simulink model "CM010A_GmT1xxMcuCfg"  (R2013b)
settings: Solver=FixedStepDiscrete  SolverMode=SingleTasking  StartTime=0.0  StopTime=0.05  RelTol=1e-3
undefined symbols (not defined in the file): BATTVLTGSCAGFAC_ULS_F32, BATTVLTGSWD1SCAGFAC_ULS_F32, BATTVLTGSWD2SCAGFAC_ULS_F32, sigbuilder_block
libraries: CM010A_GmT1xxMcuCfg_ModelLibrary x68, simulink x31
(part 1 of 3)
settings Model: Creator=nz3zln  LastModifiedBy=wzvp6q
settings SolverCC: AutoInsertRateTranBlk=on
settings DataIOCC: SignalLoggingSaveFormat=ModelDataLogs
settings OptimizationCC: ExpressionDepthLimit=2147483647
settings DebuggingCC: FcnCallInpInsideContextMsg=UseLocalSettings  FrameProcessingCompatibilityMsg=error  StateNameClashWarn=warning
settings GRTTargetCC: CodeReplacementLibrary=C89/C90 (ANSI)  CombineOutputUpdateFcns=off  GRTInterface=on

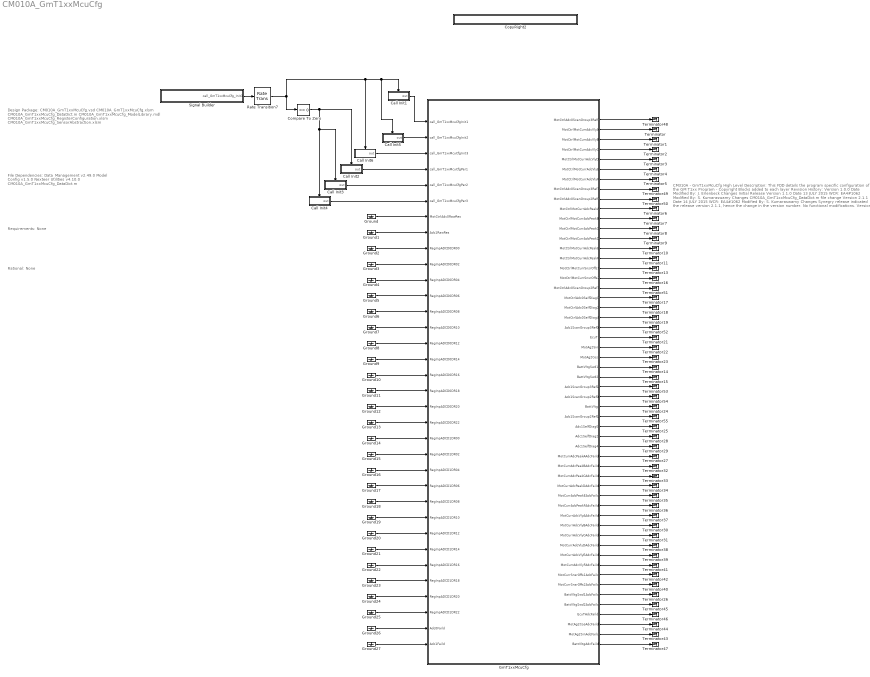
== system CM010A_GmT1xxMcuCfg ==
  note: File Dependencies:
      |
      | Data_Management v2.49.0
      | Model Config v1.5.0
      | Nexteer Utilities v4.10.0
      | CM010A_GmT1xxMcuCfg_DataDict.m
  note: CM310A - GmT1xxMcuCfg
      |
      | High Level Description:
      | This FDD details the program specific configuration of the GM T1xx Program
      |  - Copyright Blocks added to each layer
      |
      | Revision History:
      |
      | Version		1.0.0
      | Date
      | Modified By: 	J. Erlenbeck
      | Changes		Initial Release
      |
      | Version		1.1.0
      | Date 		13 JULY 2015
      | WCR:		EA4#1062
      | Modified By: 	S. Kumaraswamy
      | Changes		CM010A_GmT1xxMcuCfg_DataDict.m file change
      |
      | Version		2.1.1
      | Date 		14 JULY 2015
      | WCR:		EA4#1062
      | Modified By: 	S. Kumaraswamy
      | Changes		Synegry release indicated the release version 2.1.1, hence the
      | 			change in the version number. No functional modifications.
      |
      | Version		2.2.0
      | Date 		15 JULY 2015
      | WCR:		EA4#1109
      | Modified By: 	K. Patel
      | Changes		Motor Ag1 SPI DMA Trigger added to "CM010A_GmT1xxMcuCfg.xlsm"
      | Note: Timing vsd file need to be updated- current rev of FDD is not aligned with .vsd
      |
      |
      | Version		3.0.0
      | Date 		25JAN16
      | WCR:		EA4#3444
      | Modified By: 	Erlenbeck
      | Changes		Added GmT1xxMcuCfgPer3 to handle Adc failures
      |
      |
      | Version		3.3.0
      | Date 		07Jun16
      | WCR:		EA4#5916
      | Modified By: 	G. McCann
      | Changes		Add reference voltage read at start and end of Scan Groups 2 & 3
      |
      |
      | Version		3.4.0
      | Date 		13Sept16
      | WCR:		EA4#5916
      | Modified By: 	G. McCann
      | Changes		Removed MotCtrlAdc0DynRef and Adc1DynRef
      | 			Added NTCs in CM010A_GmT1xxMcuCfg.xlsm
      |
      |
      | Version		3.5.0
      | Date 		05Dec16
      | WCR:		EA4#8737
      | Modified By: 	G. McCann
      | Changes		No Model changes.
      | 			- Changed PwrTurnOffCtrl from PORT_PIN_LEVEL_HIGH to PORT_PIN_LEVEL_LOW
      | 			in CM010A_GmT1xxMcuCfg_PortConfig.xlsm
      | 			- Several changes to CM010A_GmT1xxMcuCfg_PortConfig.xlsm marked in red.
  note: Requirements:
      |
      | None
  note: Rational:
      |
      | None
  note: Design Package:
      |
      | CM010A_GmT1xxMcuCfg.vsd
      | CM010A_GmT1xxMcuCfg.xlsm
      | CM010A_GmT1xxMcuCfg_DataDict.m
      | CM010A_GmT1xxMcuCfg_ModelLibrary.mdl
      | CM010A_GmT1xxMcuCfg_RegisterConfiguration.xlsm
      | CM010A_GmT1xxMcuCfg_SensorAbstraction.xlsm
  Call Init1 : Subsystem  TreatAsAtomicUnit=on
  Call Init2 : Subsystem  TreatAsAtomicUnit=on
  Call Init3 : Subsystem  TreatAsAtomicUnit=on
  Call Init4 : Subsystem  TreatAsAtomicUnit=on
  Call Init5 : Subsystem  TreatAsAtomicUnit=on
  Call Init6 : Subsystem  TreatAsAtomicUnit=on
  Compare To Zero : simulink/Logic and Bit Operations/Compare To Zero  relop===  OutDataTypeStr=uint8
  CopyRight2 : Subsystem  Description=|  mask(Copyright Information){none=on}
      | Copyright info block.                                               
      |                                                                     
      | Place copyright information at the top of every subsystem in design.
      mask prompts: none "No parameters"
      mask help: Place copyright information at the top of every subsystem in design.
      mask Display:
      | NxtrConf = 'Nexteer Confidential';
      | 
      | sys = bdroot; %handle for the current model ("system")
      | first = get_param(sys,'Created');
      | first = first(end-3:end);  %year is last four digits
      | 
      | last = get_param(sys,'LastModifiedDate');
      | if isempty(last)
      |     last = datestr(now,'yyyy');
      | else
      |     last = last(end-3:end);
      | end
      | 
      | if strcmp(first,last)
      |     fprintf('%s -- Copyright %s Nexteer',NxtrConf,first)
      | else
      |     fprintf('%s -- %s%s- %s Nexteer',NxtrConf,char(169),first,last)
      | end
  GmT1xxMcuCfg : Subsystem
  Ground{,1..27} (28 alike) : Ground
  Rate Transition7 : RateTransition
  Signal Builder : Subsystem  Tag=STV Subsys  RequirementInfo={} %GIDa_2822100e_29fa_4197_9ccc_01864625f252  LoadFcn=sigbuilder_block('load');  StartFcn=sigbuilder_block('start');  StopFcn=sigbuilder_block('stop');  ClipboardFcn=sigbuilder_block('clipboard');  mask(Sigbuilder block){}
      mask help: Simulink:masks:SigbuilderBlock_MD
      mask init:
      | if ~strcmp(get_param(bdroot(gcbh),'SimulationStatus'),'stopped') tuvar = sigbuilder_block('maskInit'); end
      settings: CopyFcn=sigbuilder_block('copy');  DeleteFcn=sigbuilder_block('delete');  ModelCloseFcn=sigbuilder_block('modelClose');  PreSaveFcn=sigbuilder_block('preSave');  PauseFcn=sigbuilder_block('pause');  ContinueFcn=sigbuilder_block('continue');  NameChangeFcn=sigbuilder_block('namechange');  OpenFcn=sigbuilder_block('open',[61.5 32.25 865.5 462.75 ]);  CloseFcn=sigbuilder_block('close');
      mask Display: plot(0, 0, 100, 100,[2, 2, 32, 32, 2], [68, 8, 8, 68, 68],[32, 2], [38, 38], [32, 19, 2],[53, 60, 44], [32, 17, 17, 2],[16, 16, 31, 31]);txt = getActiveGroup(gcbh);text(2, 100, txt,'verticalAlignment', 'top');
  Terminator{,1..11,13..19,21..55} (54 alike) : Terminator
  wires:
  Signal Builder/1(call_GmT1xxMcuCfg_Init1) -> Rate Transition7/1
  Call Init1/1(out) -> GmT1xxMcuCfg/1(call_GmT1xxMcuCfgInit1)
  Rate Transition7/1 -> Compare To Zero/1, Call Init5/Enable, Call Init1/Enable, Call Init6/Enable
  Call Init2/1(out) -> GmT1xxMcuCfg/4(call_GmT1xxMcuCfgPer1)
  Call Init3/1(out) -> GmT1xxMcuCfg/5(call_GmT1xxMcuCfgPer2)
  Compare To Zero/1 -> Call Init4/Enable, Call Init3/Enable, Call Init2/Enable
  GmT1xxMcuCfg/2(MotCtrlMotCurrAdcVlyA) -> Terminator/1
  GmT1xxMcuCfg/3(MotCtrlMotCurrAdcVlyB) -> Terminator1/1
  GmT1xxMcuCfg/4(MotCtrlMotCurrAdcVlyC) -> Terminator2/1
  GmT1xxMcuCfg/5(MotCtrlMotCurrAdcVlyD) -> Terminator3/1
  GmT1xxMcuCfg/6(MotCtrlMotCurrAdcVlyE) -> Terminator4/1
  GmT1xxMcuCfg/7(MotCtrlMotCurrAdcVlyF) -> Terminator5/1
  GmT1xxMcuCfg/10(MotCtrlMotCurrAdcPeakA) -> Terminator6/1
  GmT1xxMcuCfg/11(MotCtrlMotCurrAdcPeakB) -> Terminator7/1
  GmT1xxMcuCfg/12(MotCtrlMotCurrAdcPeakC) -> Terminator8/1
  GmT1xxMcuCfg/13(MotCtrlMotCurrAdcPeakD) -> Terminator9/1
  GmT1xxMcuCfg/14(MotCtrlMotCurrAdcPeakE) -> Terminator10/1
  GmT1xxMcuCfg/15(MotCtrlMotCurrAdcPeakF) -> Terminator11/1
  GmT1xxMcuCfg/16(MotCtrlMotCurrSnsrOffs1) -> Terminator13/1
  GmT1xxMcuCfg/17(MotCtrlMotCurrSnsrOffs2) -> Terminator16/1
  GmT1xxMcuCfg/19(MotCtrlAdc0SelfDiag0) -> Terminator17/1
  GmT1xxMcuCfg/20(MotCtrlAdc0SelfDiag2) -> Terminator18/1
  GmT1xxMcuCfg/21(MotCtrlAdc0SelfDiag4) -> Terminator19/1
  GmT1xxMcuCfg/23(EcuT) -> Terminator21/1
  GmT1xxMcuCfg/24(MotAg2Sin) -> Terminator22/1
  GmT1xxMcuCfg/25(MotAg2Cos) -> Terminator23/1
  GmT1xxMcuCfg/26(BattVltgSwd1) -> Terminator14/1
  GmT1xxMcuCfg/27(BattVltgSwd2) -> Terminator15/1
  GmT1xxMcuCfg/30(BattVltg) -> Terminator24/1
  GmT1xxMcuCfg/32(Adc1SelfDiag0) -> Terminator25/1
  GmT1xxMcuCfg/33(Adc1SelfDiag2) -> Terminator28/1
  GmT1xxMcuCfg/34(Adc1SelfDiag4) -> Terminator29/1
  Ground23/1 -> GmT1xxMcuCfg/30(RegInpADCD1DR18)
  Ground20/1 -> GmT1xxMcuCfg/27(RegInpADCD1DR12)
  Ground21/1 -> GmT1xxMcuCfg/28(RegInpADCD1DR14)
  Ground16/1 -> GmT1xxMcuCfg/23(RegInpADCD1DR04)
  Ground22/1 -> GmT1xxMcuCfg/29(RegInpADCD1DR16)
  Ground19/1 -> GmT1xxMcuCfg/26(RegInpADCD1DR10)
  Ground17/1 -> GmT1xxMcuCfg/24(RegInpADCD1DR06)
  Ground18/1 -> GmT1xxMcuCfg/25(RegInpADCD1DR08)
  Ground6/1 -> GmT1xxMcuCfg/13(RegInpADCD0DR08)
  Ground1/1 -> GmT1xxMcuCfg/8(Adc1RawRes)
  Ground4/1 -> GmT1xxMcuCfg/11(RegInpADCD0DR04)
  Ground5/1 -> GmT1xxMcuCfg/12(RegInpADCD0DR06)
  Ground3/1 -> GmT1xxMcuCfg/10(RegInpADCD0DR02)
  Ground2/1 -> GmT1xxMcuCfg/9(RegInpADCD0DR00)
  Ground7/1 -> GmT1xxMcuCfg/14(RegInpADCD0DR10)
  Ground12/1 -> GmT1xxMcuCfg/19(RegInpADCD0DR20)
  Ground11/1 -> GmT1xxMcuCfg/18(RegInpADCD0DR18)
  Ground10/1 -> GmT1xxMcuCfg/17(RegInpADCD0DR16)
  Ground9/1 -> GmT1xxMcuCfg/16(RegInpADCD0DR14)
  Ground13/1 -> GmT1xxMcuCfg/20(RegInpADCD0DR22)
  Ground8/1 -> GmT1xxMcuCfg/15(RegInpADCD0DR12)
  Ground15/1 -> GmT1xxMcuCfg/22(RegInpADCD1DR02)
  Ground14/1 -> GmT1xxMcuCfg/21(RegInpADCD1DR00)
  Ground24/1 -> GmT1xxMcuCfg/31(RegInpADCD1DR20)
  Ground25/1 -> GmT1xxMcuCfg/32(RegInpADCD1DR22)
  Ground/1 -> GmT1xxMcuCfg/7(MotCtrlAdc0RawRes)
  GmT1xxMcuCfg/35(MotCurrAdcPeakAAdcFaild) -> Terminator27/1
  GmT1xxMcuCfg/36(MotCurrAdcPeakBAdcFaild) -> Terminator32/1
  GmT1xxMcuCfg/37(MotCurrAdcPeakCAdcFaild) -> Terminator33/1
  GmT1xxMcuCfg/38(MotCurrAdcPeakDAdcFaild) -> Terminator34/1
  GmT1xxMcuCfg/39(MotCurrAdcPeakEAdcFaild) -> Terminator35/1
  GmT1xxMcuCfg/40(MotCurrAdcPeakFAdcFaild) -> Terminator36/1
  GmT1xxMcuCfg/41(MotCurrAdcVlyAAdcFaild) -> Terminator37/1
  GmT1xxMcuCfg/42(MotCurrAdcVlyBAdcFaild) -> Terminator30/1
  GmT1xxMcuCfg/43(MotCurrAdcVlyCAdcFaild) -> Terminator31/1
  GmT1xxMcuCfg/44(MotCurrAdcVlyDAdcFaild) -> Terminator38/1
  GmT1xxMcuCfg/45(MotCurrAdcVlyEAdcFaild) -> Terminator39/1
  GmT1xxMcuCfg/46(MotCurrAdcVlyFAdcFaild) -> Terminator41/1
  GmT1xxMcuCfg/47(MotCurrSnsrOffs1AdcFaild) -> Terminator42/1
  GmT1xxMcuCfg/48(MotCurrSnsrOffs2AdcFaild) -> Terminator40/1
  GmT1xxMcuCfg/49(BattVltgSwd1AdcFaild) -> Terminator26/1
  GmT1xxMcuCfg/50(BattVltgSwd2AdcFaild) -> Terminator45/1
  GmT1xxMcuCfg/51(EcuTAdcFaild) -> Terminator46/1
  GmT1xxMcuCfg/52(MotAg2CosAdcFaild) -> Terminator44/1
  GmT1xxMcuCfg/53(MotAg2SinAdcFaild) -> Terminator43/1
  Ground26/1 -> GmT1xxMcuCfg/33(Adc0Faild)
  Ground27/1 -> GmT1xxMcuCfg/34(Adc1Faild)
  Call Init4/1(out) -> GmT1xxMcuCfg/6(call_GmT1xxMcuCfgPer3)
  Call Init5/1(out) -> GmT1xxMcuCfg/2(call_GmT1xxMcuCfgInit2)
  Call Init6/1(out) -> GmT1xxMcuCfg/3(call_GmT1xxMcuCfgInit3)
  GmT1xxMcuCfg/54(BattVltgAdcFaild) -> Terminator47/1
  GmT1xxMcuCfg/1(MotCtrlAdc0ScanGroup3Ref0) -> Terminator48/1
  GmT1xxMcuCfg/8(MotCtrlAdc0ScanGroup3Ref1) -> Terminator49/1
  GmT1xxMcuCfg/9(MotCtrlAdc0ScanGroup2Ref0) -> Terminator50/1
  GmT1xxMcuCfg/18(MotCtrlAdc0ScanGroup2Ref1) -> Terminator51/1
  GmT1xxMcuCfg/22(Adc1ScanGroup3Ref0) -> Terminator52/1
  GmT1xxMcuCfg/28(Adc1ScanGroup3Ref1) -> Terminator53/1
  GmT1xxMcuCfg/29(Adc1ScanGroup2Ref0) -> Terminator54/1
  GmT1xxMcuCfg/31(Adc1ScanGroup2Ref1) -> Terminator55/1

== system CM010A_GmT1xxMcuCfg/Call Init1 ==
  Enable : EnablePort
  Function Call Trigger : simulink/Ports & Subsystems/Function-Call Generator  RequirementInfo="{'linktype_rmi_doors' '000089e3 (/E-STEER_New/System Specification Documents/Core Specs/Subsystem Specs/System Functions FDD/SF-46  Gross Cross Check)' '#211' 'true' '3.1-1 The GCC function shall monitor every posted output motor comm' '' ; 'linktype_rmi_doors' '000089e3 (/E-STEER_New/System Specification Documents/Core Specs/Subsystem Specs/System Functions FDD/SF-46  Gross Cross Check)' '#182' 'true' '3.2.2-1 GCC shall be executed at a 0.002 second loop time.' '' } %GIDa_ff755a2e_49d1_45f7_8591_3ce0ef475338"  sample_time=0.0005  numberOfIterations=1
  out : Outport
  wires:
  Function Call Trigger/1 -> out/1

== system CM010A_GmT1xxMcuCfg/Call Init2 ==
  Enable : EnablePort
  Function Call Trigger : simulink/Ports & Subsystems/Function-Call Generator  RequirementInfo="{'linktype_rmi_doors' '000089e3 (/E-STEER_New/System Specification Documents/Core Specs/Subsystem Specs/System Functions FDD/SF-46  Gross Cross Check)' '#211' 'true' '3.1-1 The GCC function shall monitor every posted output motor comm' '' ; 'linktype_rmi_doors' '000089e3 (/E-STEER_New/System Specification Documents/Core Specs/Subsystem Specs/System Functions FDD/SF-46  Gross Cross Check)' '#182' 'true' '3.2.2-1 GCC shall be executed at a 0.002 second loop time.' '' } %GIDa_ba5be832_aeac_40ae_ae53_3fd25198366e"  sample_time=0.0005  numberOfIterations=1
  out : Outport
  wires:
  Function Call Trigger/1 -> out/1

== system CM010A_GmT1xxMcuCfg/Call Init3 ==
  Enable : EnablePort
  Function Call Trigger : simulink/Ports & Subsystems/Function-Call Generator  RequirementInfo="{'linktype_rmi_doors' '000089e3 (/E-STEER_New/System Specification Documents/Core Specs/Subsystem Specs/System Functions FDD/SF-46  Gross Cross Check)' '#211' 'true' '3.1-1 The GCC function shall monitor every posted output motor comm' '' ; 'linktype_rmi_doors' '000089e3 (/E-STEER_New/System Specification Documents/Core Specs/Subsystem Specs/System Functions FDD/SF-46  Gross Cross Check)' '#182' 'true' '3.2.2-1 GCC shall be executed at a 0.002 second loop time.' '' } %GIDa_bf682727_f4b1_4f52_ae72_c6f6d8d412d7"  sample_time=0.002  numberOfIterations=1
  out : Outport
  wires:
  Function Call Trigger/1 -> out/1

== system CM010A_GmT1xxMcuCfg/Call Init4 ==
  Enable : EnablePort
  Function Call Trigger : simulink/Ports & Subsystems/Function-Call Generator  RequirementInfo="{'linktype_rmi_doors' '000089e3 (/E-STEER_New/System Specification Documents/Core Specs/Subsystem Specs/System Functions FDD/SF-46  Gross Cross Check)' '#211' 'true' '3.1-1 The GCC function shall monitor every posted output motor comm' '' ; 'linktype_rmi_doors' '000089e3 (/E-STEER_New/System Specification Documents/Core Specs/Subsystem Specs/System Functions FDD/SF-46  Gross Cross Check)' '#182' 'true' '3.2.2-1 GCC shall be executed at a 0.002 second loop time.' '' } %GIDa_39162fcb_260a_4191_9640_bf2fa4fe87e2"  sample_time=0.002  numberOfIterations=1
  out : Outport
  wires:
  Function Call Trigger/1 -> out/1

== system CM010A_GmT1xxMcuCfg/Call Init5 ==
  Enable : EnablePort
  Function Call Trigger : simulink/Ports & Subsystems/Function-Call Generator  RequirementInfo="{'linktype_rmi_doors' '000089e3 (/E-STEER_New/System Specification Documents/Core Specs/Subsystem Specs/System Functions FDD/SF-46  Gross Cross Check)' '#211' 'true' '3.1-1 The GCC function shall monitor every posted output motor comm' '' ; 'linktype_rmi_doors' '000089e3 (/E-STEER_New/System Specification Documents/Core Specs/Subsystem Specs/System Functions FDD/SF-46  Gross Cross Check)' '#182' 'true' '3.2.2-1 GCC shall be executed at a 0.002 second loop time.' '' } %GIDa_52b82f2d_d21e_4ccf_9b87_2b660c433421"  sample_time=0.0005  numberOfIterations=1
  out : Outport
  wires:
  Function Call Trigger/1 -> out/1

== system CM010A_GmT1xxMcuCfg/Call Init6 ==
  Enable : EnablePort
  Function Call Trigger : simulink/Ports & Subsystems/Function-Call Generator  RequirementInfo="{'linktype_rmi_doors' '000089e3 (/E-STEER_New/System Specification Documents/Core Specs/Subsystem Specs/System Functions FDD/SF-46  Gross Cross Check)' '#211' 'true' '3.1-1 The GCC function shall monitor every posted output motor comm' '' ; 'linktype_rmi_doors' '000089e3 (/E-STEER_New/System Specification Documents/Core Specs/Subsystem Specs/System Functions FDD/SF-46  Gross Cross Check)' '#182' 'true' '3.2.2-1 GCC shall be executed at a 0.002 second loop time.' '' } %GIDa_40b20fc1_ef82_4ce8_9bb2_77ecb7477d85"  sample_time=0.0005  numberOfIterations=1
  out : Outport
  wires:
  Function Call Trigger/1 -> out/1

== system CM010A_GmT1xxMcuCfg/CopyRight2 ==

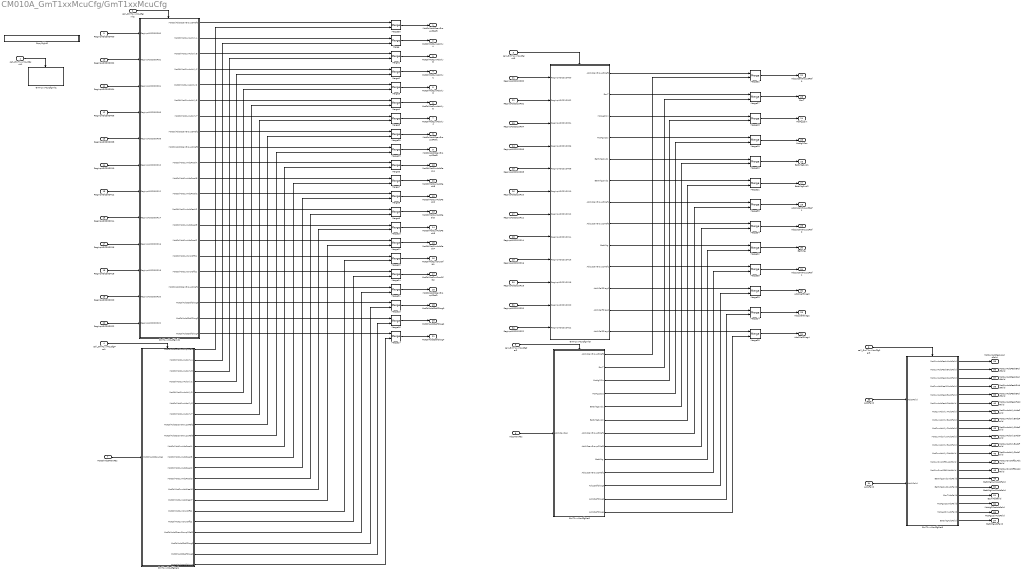
== system CM010A_GmT1xxMcuCfg/GmT1xxMcuCfg ==
  call_GmT1xxMcuCfgInit1 : Inport
  call_GmT1xxMcuCfgInit2 : Inport  Port=2
  call_GmT1xxMcuCfgInit3 : Inport  Port=3
  call_GmT1xxMcuCfgPer1 : Inport  Port=4
  call_GmT1xxMcuCfgPer2 : Inport  Port=5
  call_GmT1xxMcuCfgPer3 : Inport  Port=6
  MotCtrlAdc0RawRes : Inport  Port=7
  Adc1RawRes : Inport  Port=8
  RegInpADCD0DR00 : Inport  Port=9  OutDataTypeStr=uint32
  RegInpADCD0DR02 : Inport  Port=10  OutDataTypeStr=uint32
  RegInpADCD0DR04 : Inport  Port=11  OutDataTypeStr=uint32
  RegInpADCD0DR06 : Inport  Port=12  OutDataTypeStr=uint32
  RegInpADCD0DR08 : Inport  Port=13  OutDataTypeStr=uint32
  RegInpADCD0DR10 : Inport  Port=14  OutDataTypeStr=uint32
  RegInpADCD0DR12 : Inport  Port=15  OutDataTypeStr=uint32
  RegInpADCD0DR14 : Inport  Port=16  OutDataTypeStr=uint32
  RegInpADCD0DR16 : Inport  Port=17  OutDataTypeStr=uint32
  RegInpADCD0DR18 : Inport  Port=18  OutDataTypeStr=uint32
  RegInpADCD0DR20 : Inport  Port=19  OutDataTypeStr=uint32
  RegInpADCD0DR22 : Inport  Port=20  OutDataTypeStr=uint32
  RegInpADCD1DR00 : Inport  Port=21  OutDataTypeStr=uint32
  RegInpADCD1DR02 : Inport  Port=22  OutDataTypeStr=uint32
  RegInpADCD1DR04 : Inport  Port=23  OutDataTypeStr=uint32
  RegInpADCD1DR06 : Inport  Port=24  OutDataTypeStr=uint32
  RegInpADCD1DR08 : Inport  Port=25  OutDataTypeStr=uint32
  RegInpADCD1DR10 : Inport  Port=26  OutDataTypeStr=uint32
  RegInpADCD1DR12 : Inport  Port=27  OutDataTypeStr=uint32
  RegInpADCD1DR14 : Inport  Port=28  OutDataTypeStr=uint32
  RegInpADCD1DR16 : Inport  Port=29  OutDataTypeStr=uint32
  RegInpADCD1DR18 : Inport  Port=30  OutDataTypeStr=uint32
  RegInpADCD1DR20 : Inport  Port=31  OutDataTypeStr=uint32
  RegInpADCD1DR22 : Inport  Port=32  OutDataTypeStr=uint32
  Adc0Faild : Inport  Port=33
  Adc1Faild : Inport  Port=34
  CopyRight2 : Subsystem  Description=|  mask(Copyright Information){none=on}
      | Copyright info block.                                               
      |                                                                     
      | Place copyright information at the top of every subsystem in design.
      mask prompts: none "No parameters"
      mask help: Place copyright information at the top of every subsystem in design.
      mask Display:
      | NxtrConf = 'Nexteer Confidential';
      | 
      | sys = bdroot; %handle for the current model ("system")
      | first = get_param(sys,'Created');
      | first = first(end-3:end);  %year is last four digits
      | 
      | last = get_param(sys,'LastModifiedDate');
      | if isempty(last)
      |     last = datestr(now,'yyyy');
      | else
      |     last = last(end-3:end);
      | end
      | 
      | if strcmp(first,last)
      |     fprintf('%s -- Copyright %s Nexteer',NxtrConf,first)
      | else
      |     fprintf('%s -- %s%s- %s Nexteer',NxtrConf,char(169),first,last)
      | end
  GmT1xxMcuCfgInit1 : Subsystem
  GmT1xxMcuCfgInit2 : Subsystem
  GmT1xxMcuCfgInit3 : Subsystem
  GmT1xxMcuCfgPer1 : Subsystem  RequirementInfo={'linktype_rmi_doors' '0000c472 (/ESG Group/FDD Module Requirements/EA4 Specific/CM300A_Adc0CfgAndUse)' '#CM300A_76' 'true' 'REQ: CM300A_76' '' ; 'linktype_rmi_doors' '0000c472 (/ESG Group/FDD Module Requirements/EA4 Specific/CM300A_Adc0CfgAndUse)' '#CM300A_81' 'true' 'REQ: CM300A_81' '' ; 'linktype_rmi_doors' '0000c472 (/ESG Group/FDD Module Requirements/EA4 Specific/CM300A_Adc0CfgAndUse)' '#CM300A_82' 'true' 'REQ: CM300A_82' '' } %GIDa_873a1ca9_93ed_4591_b882_6d7fd3820ab2
      settings: AttributesFormatString=Priority: %<Priority>
  GmT1xxMcuCfgPer2 : Subsystem  RequirementInfo={'linktype_rmi_doors' '0000c472 (/ESG Group/FDD Module Requirements/EA4 Specific/CM300A_Adc0CfgAndUse)' '#CM300A_76' 'true' 'REQ: CM300A_76' '' ; 'linktype_rmi_doors' '0000c472 (/ESG Group/FDD Module Requirements/EA4 Specific/CM300A_Adc0CfgAndUse)' '#CM300A_81' 'true' 'REQ: CM300A_81' '' ; 'linktype_rmi_doors' '0000c472 (/ESG Group/FDD Module Requirements/EA4 Specific/CM300A_Adc0CfgAndUse)' '#CM300A_82' 'true' 'REQ: CM300A_82' '' } %GIDa_f8eec309_27b4_4df0_b18c_c2951f94362c
      settings: AttributesFormatString=Priority: %<Priority>
  GmT1xxMcuCfgPer3 : Subsystem  RequirementInfo={'linktype_rmi_doors' '0000c472 (/ESG Group/FDD Module Requirements/EA4 Specific/CM300A_Adc0CfgAndUse)' '#CM300A_76' 'true' 'REQ: CM300A_76' '' ; 'linktype_rmi_doors' '0000c472 (/ESG Group/FDD Module Requirements/EA4 Specific/CM300A_Adc0CfgAndUse)' '#CM300A_81' 'true' 'REQ: CM300A_81' '' ; 'linktype_rmi_doors' '0000c472 (/ESG Group/FDD Module Requirements/EA4 Specific/CM300A_Adc0CfgAndUse)' '#CM300A_82' 'true' 'REQ: CM300A_82' '' } %GIDa_f61b09d0_e9f4_4379_bee3_c878705b543d
      settings: AttributesFormatString=Priority: %<Priority>
  Merge{,1..11,13..25,27..35} (34 alike) : Merge
  MotCtrlAdc0ScanGroup3Ref0 : Outport
  MotCtrlMotCurrAdcVlyA : Outport  Port=2
  MotCtrlMotCurrAdcVlyB : Outport  Port=3
  MotCtrlMotCurrAdcVlyC : Outport  Port=4
  MotCtrlMotCurrAdcVlyD : Outport  Port=5
  MotCtrlMotCurrAdcVlyE : Outport  Port=6
  MotCtrlMotCurrAdcVlyF : Outport  Port=7
  MotCtrlAdc0ScanGroup3Ref1 : Outport  Port=8
  MotCtrlAdc0ScanGroup2Ref0 : Outport  Port=9
  MotCtrlMotCurrAdcPeakA : Outport  Port=10
  MotCtrlMotCurrAdcPeakB : Outport  Port=11
  MotCtrlMotCurrAdcPeakC : Outport  Port=12
  MotCtrlMotCurrAdcPeakD : Outport  Port=13
  MotCtrlMotCurrAdcPeakE : Outport  Port=14
  MotCtrlMotCurrAdcPeakF : Outport  Port=15
  MotCtrlMotCurrSnsrOffs1 : Outport  Port=16
  MotCtrlMotCurrSnsrOffs2 : Outport  Port=17
  MotCtrlAdc0ScanGroup2Ref1 : Outport  Port=18
  MotCtrlAdc0SelfDiag0 : Outport  Port=19
  MotCtrlAdc0SelfDiag2 : Outport  Port=20
  MotCtrlAdc0SelfDiag4 : Outport  Port=21
  Adc1ScanGroup3Ref0 : Outport  Port=22
  EcuT : Outport  Port=23
  MotAg2Sin : Outport  Port=24
  MotAg2Cos : Outport  Port=25
  BattVltgSwd1 : Outport  Port=26
  BattVltgSwd2 : Outport  Port=27
  Adc1ScanGroup3Ref1 : Outport  Port=28
  Adc1ScanGroup2Ref0 : Outport  Port=29
  BattVltg : Outport  Port=30
  Adc1ScanGroup2Ref1 : Outport  Port=31
  Adc1SelfDiag0 : Outport  Port=32
  Adc1SelfDiag2 : Outport  Port=33
  Adc1SelfDiag4 : Outport  Port=34
  MotCurrAdcPeakAAdcFaild : Outport  Port=35
  MotCurrAdcPeakBAdcFaild : Outport  Port=36
  MotCurrAdcPeakCAdcFaild : Outport  Port=37
  MotCurrAdcPeakDAdcFaild : Outport  Port=38
  MotCurrAdcPeakEAdcFaild : Outport  Port=39
  MotCurrAdcPeakFAdcFaild : Outport  Port=40
  MotCurrAdcVlyAAdcFaild : Outport  Port=41
  MotCurrAdcVlyBAdcFaild : Outport  Port=42
  MotCurrAdcVlyCAdcFaild : Outport  Port=43
  MotCurrAdcVlyDAdcFaild : Outport  Port=44
  MotCurrAdcVlyEAdcFaild : Outport  Port=45
  MotCurrAdcVlyFAdcFaild : Outport  Port=46
  MotCurrSnsrOffs1AdcFaild : Outport  Port=47
  MotCurrSnsrOffs2AdcFaild : Outport  Port=48
  BattVltgSwd1AdcFaild : Outport  Port=49
  BattVltgSwd2AdcFaild : Outport  Port=50
  EcuTAdcFaild : Outport  Port=51
  MotAg2CosAdcFaild : Outport  Port=52
  MotAg2SinAdcFaild : Outport  Port=53
  BattVltgAdcFaild : Outport  Port=54
  wires:
  call_GmT1xxMcuCfgPer1/1 -> GmT1xxMcuCfgPer1/Trigger
  call_GmT1xxMcuCfgPer2/1 -> GmT1xxMcuCfgPer2/Trigger
  GmT1xxMcuCfgInit2/2(MotCtrlMotCurrAdcVlyA) -> Merge/1
  Merge/1 -> MotCtrlMotCurrAdcVlyA/1
  GmT1xxMcuCfgInit2/3(MotCtrlMotCurrAdcVlyB) -> Merge1/1
  Merge1/1 -> MotCtrlMotCurrAdcVlyB/1
  Merge2/1 -> MotCtrlMotCurrAdcVlyC/1
  GmT1xxMcuCfgInit2/4(MotCtrlMotCurrAdcVlyC) -> Merge2/1
  GmT1xxMcuCfgInit2/5(MotCtrlMotCurrAdcVlyD) -> Merge3/1
  Merge3/1 -> MotCtrlMotCurrAdcVlyD/1
  GmT1xxMcuCfgInit2/6(MotCtrlMotCurrAdcVlyE) -> Merge4/1
  GmT1xxMcuCfgInit2/7(MotCtrlMotCurrAdcVlyF) -> Merge5/1
  Merge4/1 -> MotCtrlMotCurrAdcVlyE/1
  Merge5/1 -> MotCtrlMotCurrAdcVlyF/1
  GmT1xxMcuCfgInit2/10(MotCtrlMotCurrAdcPeakA) -> Merge6/1
  Merge6/1 -> MotCtrlMotCurrAdcPeakA/1
  GmT1xxMcuCfgInit2/11(MotCtrlMotCurrAdcPeakB) -> Merge7/1
  GmT1xxMcuCfgInit2/12(MotCtrlMotCurrAdcPeakC) -> Merge8/1
  GmT1xxMcuCfgInit2/13(MotCtrlMotCurrAdcPeakD) -> Merge9/1
  GmT1xxMcuCfgInit2/14(MotCtrlMotCurrAdcPeakE) -> Merge10/1
  GmT1xxMcuCfgInit2/15(MotCtrlMotCurrAdcPeakF) -> Merge11/1
  GmT1xxMcuCfgInit2/16(MotCtrlMotCurrSnsrOffs1) -> Merge13/1
  Merge7/1 -> MotCtrlMotCurrAdcPeakB/1
  Merge8/1 -> MotCtrlMotCurrAdcPeakC/1
  Merge9/1 -> MotCtrlMotCurrAdcPeakD/1
  Merge10/1 -> MotCtrlMotCurrAdcPeakE/1
  Merge11/1 -> MotCtrlMotCurrAdcPeakF/1
  Merge13/1 -> MotCtrlMotCurrSnsrOffs1/1
  GmT1xxMcuCfgInit2/17(MotCtrlMotCurrSnsrOffs2) -> Merge14/1
  GmT1xxMcuCfgInit2/19(MotCtrlAdc0SelfDiag0) -> Merge15/1
  GmT1xxMcuCfgInit2/20(MotCtrlAdc0SelfDiag2) -> Merge16/1
  GmT1xxMcuCfgInit2/21(MotCtrlAdc0SelfDiag4) -> Merge17/1
  Merge14/1 -> MotCtrlMotCurrSnsrOffs2/1
  Merge15/1 -> MotCtrlAdc0SelfDiag0/1
  Merge16/1 -> MotCtrlAdc0SelfDiag2/1
  Merge17/1 -> MotCtrlAdc0SelfDiag4/1
  Merge27/1 -> EcuT/1
  Merge18/1 -> MotAg2Sin/1
  Merge19/1 -> MotAg2Cos/1
  Merge20/1 -> BattVltgSwd1/1
  Merge21/1 -> BattVltgSwd2/1
  Merge22/1 -> BattVltg/1
  Merge23/1 -> Adc1SelfDiag0/1
  Merge24/1 -> Adc1SelfDiag2/1
  Merge25/1 -> Adc1SelfDiag4/1
  RegInpADCD1DR00/1 -> GmT1xxMcuCfgInit3/1(RegInpADCD1DR00)
  RegInpADCD1DR02/1 -> GmT1xxMcuCfgInit3/2(RegInpADCD1DR02)
  RegInpADCD1DR04/1 -> GmT1xxMcuCfgInit3/3(RegInpADCD1DR04)
  RegInpADCD1DR06/1 -> GmT1xxMcuCfgInit3/4(RegInpADCD1DR06)
  RegInpADCD1DR08/1 -> GmT1xxMcuCfgInit3/5(RegInpADCD1DR08)
  RegInpADCD1DR10/1 -> GmT1xxMcuCfgInit3/6(RegInpADCD1DR10)
  RegInpADCD1DR12/1 -> GmT1xxMcuCfgInit3/7(RegInpADCD1DR12)
  RegInpADCD1DR14/1 -> GmT1xxMcuCfgInit3/8(RegInpADCD1DR14)
  RegInpADCD1DR16/1 -> GmT1xxMcuCfgInit3/9(RegInpADCD1DR16)
  RegInpADCD1DR18/1 -> GmT1xxMcuCfgInit3/10(RegInpADCD1DR18)
  RegInpADCD1DR20/1 -> GmT1xxMcuCfgInit3/11(RegInpADCD1DR20)
  RegInpADCD1DR22/1 -> GmT1xxMcuCfgInit3/12(RegInpADCD1DR22)
  RegInpADCD0DR00/1 -> GmT1xxMcuCfgInit2/1(RegInpADCD0DR00)
  RegInpADCD0DR02/1 -> GmT1xxMcuCfgInit2/2(RegInpADCD0DR02)
  RegInpADCD0DR04/1 -> GmT1xxMcuCfgInit2/3(RegInpADCD0DR04)
  RegInpADCD0DR06/1 -> GmT1xxMcuCfgInit2/4(RegInpADCD0DR06)
  RegInpADCD0DR08/1 -> GmT1xxMcuCfgInit2/5(RegInpADCD0DR08)
  RegInpADCD0DR10/1 -> GmT1xxMcuCfgInit2/6(RegInpADCD0DR10)
  RegInpADCD0DR12/1 -> GmT1xxMcuCfgInit2/7(RegInpADCD0DR12)
  RegInpADCD0DR14/1 -> GmT1xxMcuCfgInit2/8(RegInpADCD0DR14)
  RegInpADCD0DR16/1 -> GmT1xxMcuCfgInit2/9(RegInpADCD0DR16)
  RegInpADCD0DR18/1 -> GmT1xxMcuCfgInit2/10(RegInpADCD0DR18)
  RegInpADCD0DR20/1 -> GmT1xxMcuCfgInit2/11(RegInpADCD0DR20)
  RegInpADCD0DR22/1 -> GmT1xxMcuCfgInit2/12(RegInpADCD0DR22)
  GmT1xxMcuCfgPer1/2(MotCtrlMotCurrAdcVlyA) -> Merge/2
  GmT1xxMcuCfgPer1/3(MotCtrlMotCurrAdcVlyB) -> Merge1/2
  GmT1xxMcuCfgPer1/4(MotCtrlMotCurrAdcVlyC) -> Merge2/2
  GmT1xxMcuCfgPer1/5(MotCtrlMotCurrAdcVlyD) -> Merge3/2
  GmT1xxMcuCfgPer1/6(MotCtrlMotCurrAdcVlyE) -> Merge4/2
  GmT1xxMcuCfgPer1/7(MotCtrlMotCurrAdcVlyF) -> Merge5/2
  GmT1xxMcuCfgPer1/10(MotCtrlMotCurrAdcPeakA) -> Merge6/2
  GmT1xxMcuCfgPer1/11(MotCtrlMotCurrAdcPeakB) -> Merge7/2
  GmT1xxMcuCfgPer1/12(MotCtrlMotCurrAdcPeakC) -> Merge8/2
  GmT1xxMcuCfgPer1/13(MotCtrlMotCurrAdcPeakD) -> Merge9/2
  GmT1xxMcuCfgPer1/14(MotCtrlMotCurrAdcPeakE) -> Merge10/2
  GmT1xxMcuCfgPer1/15(MotCtrlMotCurrAdcPeakF) -> Merge11/2
  GmT1xxMcuCfgPer1/16(MotCtrlMotCurrSnsrOffs1) -> Merge13/2
  GmT1xxMcuCfgPer1/17(MotCtrlMotCurrSnsrOffs2) -> Merge14/2
  GmT1xxMcuCfgPer1/19(MotCtrlAdc0SelfDiag0) -> Merge15/2
  GmT1xxMcuCfgPer1/20(MotCtrlAdc0SelfDiag2) -> Merge16/2
  GmT1xxMcuCfgPer1/21(MotCtrlAdc0SelfDiag4) -> Merge17/2
  call_GmT1xxMcuCfgInit1/1 -> GmT1xxMcuCfgInit1/Trigger
  GmT1xxMcuCfgInit3/2(EcuT) -> Merge27/1
  GmT1xxMcuCfgInit3/3(MotAg2Sin) -> Merge18/1
  GmT1xxMcuCfgInit3/4(MotAg2Cos) -> Merge19/1
  GmT1xxMcuCfgInit3/5(BattVltgSwd1) -> Merge20/1
  GmT1xxMcuCfgInit3/6(BattVltgSwd2) -> Merge21/1
  GmT1xxMcuCfgInit3/9(BattVltg) -> Merge22/1
  GmT1xxMcuCfgInit3/11(Adc1SelfDiag0) -> Merge23/1
  GmT1xxMcuCfgInit3/12(Adc1SelfDiag2) -> Merge24/1
  GmT1xxMcuCfgInit3/13(Adc1SelfDiag4) -> Merge25/1
  GmT1xxMcuCfgPer2/2(EcuT) -> Merge27/2
  GmT1xxMcuCfgPer2/3(MotAg2Sin) -> Merge18/2
  GmT1xxMcuCfgPer2/4(MotAg2Cos) -> Merge19/2
  GmT1xxMcuCfgPer2/5(BattVltgSwd1) -> Merge20/2
  GmT1xxMcuCfgPer2/6(BattVltgSwd2) -> Merge21/2
  GmT1xxMcuCfgPer2/9(BattVltg) -> Merge22/2
  GmT1xxMcuCfgPer2/11(Adc1SelfDiag0) -> Merge23/2
  GmT1xxMcuCfgPer2/12(Adc1SelfDiag2) -> Merge24/2
  GmT1xxMcuCfgPer2/13(Adc1SelfDiag4) -> Merge25/2
  MotCtrlAdc0RawRes/1 -> GmT1xxMcuCfgPer1/1(MotCtrlAdc0RawRes)
  Adc1RawRes/1 -> GmT1xxMcuCfgPer2/1(Adc1RawRes)
  call_GmT1xxMcuCfgPer3/1 -> GmT1xxMcuCfgPer3/Trigger
  Adc0Faild/1 -> GmT1xxMcuCfgPer3/1(Adc0Faild)
  Adc1Faild/1 -> GmT1xxMcuCfgPer3/2(Adc1Faild)
  GmT1xxMcuCfgPer3/1(MotCurrAdcPeakAAdcFaild) -> MotCurrAdcPeakAAdcFaild/1
  GmT1xxMcuCfgPer3/2(MotCurrAdcPeakBAdcFaild) -> MotCurrAdcPeakBAdcFaild/1
  GmT1xxMcuCfgPer3/3(MotCurrAdcPeakCAdcFaild) -> MotCurrAdcPeakCAdcFaild/1
  GmT1xxMcuCfgPer3/4(MotCurrAdcPeakDAdcFaild) -> MotCurrAdcPeakDAdcFaild/1
  GmT1xxMcuCfgPer3/5(MotCurrAdcPeakEAdcFaild) -> MotCurrAdcPeakEAdcFaild/1
  GmT1xxMcuCfgPer3/6(MotCurrAdcPeakFAdcFaild) -> MotCurrAdcPeakFAdcFaild/1
  GmT1xxMcuCfgPer3/7(MotCurrAdcVlyAAdcFaild) -> MotCurrAdcVlyAAdcFaild/1
  GmT1xxMcuCfgPer3/8(MotCurrAdcVlyBAdcFaild) -> MotCurrAdcVlyBAdcFaild/1
  GmT1xxMcuCfgPer3/9(MotCurrAdcVlyCAdcFaild) -> MotCurrAdcVlyCAdcFaild/1
  GmT1xxMcuCfgPer3/10(MotCurrAdcVlyDAdcFaild) -> MotCurrAdcVlyDAdcFaild/1
  GmT1xxMcuCfgPer3/11(MotCurrAdcVlyEAdcFaild) -> MotCurrAdcVlyEAdcFaild/1
  GmT1xxMcuCfgPer3/12(MotCurrAdcVlyFAdcFaild) -> MotCurrAdcVlyFAdcFaild/1
  GmT1xxMcuCfgPer3/13(MotCurrSnsrOffs1AdcFaild) -> MotCurrSnsrOffs1AdcFaild/1
  GmT1xxMcuCfgPer3/14(MotCurrSnsrOffs2AdcFaild) -> MotCurrSnsrOffs2AdcFaild/1
  GmT1xxMcuCfgPer3/15(BattVltgSwd1AdcFaild) -> BattVltgSwd1AdcFaild/1
  GmT1xxMcuCfgPer3/16(BattVltgSwd2AdcFaild) -> BattVltgSwd2AdcFaild/1
  GmT1xxMcuCfgPer3/17(EcuTAdcFaild) -> EcuTAdcFaild/1
  GmT1xxMcuCfgPer3/18(MotAg2CosAdcFaild) -> MotAg2CosAdcFaild/1
  GmT1xxMcuCfgPer3/19(MotAg2SinAdcFaild) -> MotAg2SinAdcFaild/1
  call_GmT1xxMcuCfgInit2/1 -> GmT1xxMcuCfgInit2/Trigger
  call_GmT1xxMcuCfgInit3/1 -> GmT1xxMcuCfgInit3/Trigger
  GmT1xxMcuCfgPer3/20(BattVltgAdcFaild) -> BattVltgAdcFaild/1
  Merge28/1 -> MotCtrlAdc0ScanGroup3Ref1/1
  Merge29/1 -> MotCtrlAdc0ScanGroup2Ref0/1
  GmT1xxMcuCfgInit2/8(MotCtrlAdc0ScanGroup3Ref1) -> Merge28/1
  GmT1xxMcuCfgInit2/9(MotCtrlAdc0ScanGroup2Ref0) -> Merge29/1
  Merge30/1 -> MotCtrlAdc0ScanGroup3Ref0/1
  GmT1xxMcuCfgInit2/1(MotCtrlAdc0ScanGroup3Ref0) -> Merge30/1
  Merge31/1 -> MotCtrlAdc0ScanGroup2Ref1/1
  GmT1xxMcuCfgInit2/18(MotCtrlAdc0ScanGroup2Ref1) -> Merge31/1
  GmT1xxMcuCfgPer1/1(MotCtrlAdc0ScanGroup3Ref0) -> Merge30/2
  GmT1xxMcuCfgPer1/8(MotCtrlAdc0ScanGroup3Ref1) -> Merge28/2
  GmT1xxMcuCfgPer1/9(MotCtrlAdc0ScanGroup2Ref0) -> Merge29/2
  GmT1xxMcuCfgPer1/18(MotCtrlAdc0ScanGroup2Ref1) -> Merge31/2
  Merge32/1 -> Adc1ScanGroup3Ref0/1
  GmT1xxMcuCfgInit3/1(Adc1ScanGroup3Ref0) -> Merge32/1
  GmT1xxMcuCfgInit3/8(Adc1ScanGroup2Ref0) -> Merge34/1
  GmT1xxMcuCfgInit3/7(Adc1ScanGroup3Ref1) -> Merge33/1
  Merge34/1 -> Adc1ScanGroup2Ref0/1
  Merge33/1 -> Adc1ScanGroup3Ref1/1
  GmT1xxMcuCfgInit3/10(Adc1ScanGroup2Ref1) -> Merge35/1
  Merge35/1 -> Adc1ScanGroup2Ref1/1
  GmT1xxMcuCfgPer2/1(Adc1ScanGroup3Ref0) -> Merge32/2
  GmT1xxMcuCfgPer2/7(Adc1ScanGroup3Ref1) -> Merge33/2
  GmT1xxMcuCfgPer2/8(Adc1ScanGroup2Ref0) -> Merge34/2
  GmT1xxMcuCfgPer2/10(Adc1ScanGroup2Ref1) -> Merge35/2

== system CM010A_GmT1xxMcuCfg/Signal Builder ==
  Demux : Demux  Tag=STV Demux  Outputs=1
  FromWs : FromWorkspace  Tag=STV FromWs  VariableName=tuvar  SampleTime=0
      SigBuilderData=|
      | common.afterFinalStr = 'Extrapolate'
      | common.sampleTime = 0
      | dataSet(1).timeRange = [0 0.5]
      | dataSet(1).name = 'Group 1'
      | dataSet(2).timeRange = [0 0.5]
      | dataSet(2).name = 'Group 2'
      | dataSet(3).timeRange = [0 1.2]
      | dataSet(3).name = 'Group 3'
      | dataSet(4).timeRange = [0 5]
      | dataSet(4).name = 'Group 4'
      | dataSet(5).timeRange = [0 10]
      | dataSet(5).name = 'Group 5'
      | dataSet(6).timeRange = [0 8]
      | dataSet(6).name = 'Group 6'
      | sbobj.Groups(1).Name = 'Group 1'
      | sbobj.Groups(1).Signals.Name = 'call_GmT1xxMcuCfg_Init1'
      | sbobj.Groups(1).Signals.XData = [0 0.001 0.001 0.5]
      | sbobj.Groups(1).Signals.YData = [1 1 0 0]
      | sbobj.Groups(1).TimeRange = [0 0.5]
      | sbobj.Groups(2).Name = 'Group 2'
      | sbobj.Groups(2).Signals.Name = 'call_GmT1xxMcuCfg_Init1'
      | sbobj.Groups(2).Signals.XData = [0 0.001 0.001 0.5]
      | sbobj.Groups(2).Signals.YData = [1 1 0 0]
      | sbobj.Groups(2).TimeRange = [0 0.5]
      | sbobj.Groups(3).Name = 'Group 3'
      | sbobj.Groups(3).Signals.Name = 'call_GmT1xxMcuCfg_Init1'
      | sbobj.Groups(3).Signals.XData = [0 0.001 0.001 1.2]
      | sbobj.Groups(3).Signals.YData = [1 1 0 0]
      | sbobj.Groups(3).TimeRange = [0 1.2]
      | sbobj.Groups(4).Name = 'Group 4'
      | sbobj.Groups(4).Signals.Name = 'call_GmT1xxMcuCfg_Init1'
      | sbobj.Groups(4).Signals.XData = [0 0.001 0.001 5]
      | sbobj.Groups(4).Signals.YData = [1 1 0 0]
      | sbobj.Groups(4).TimeRange = [0 5]
      | sbobj.Groups(5).Name = 'Group 5'
      | sbobj.Groups(5).Signals.Name = 'call_GmT1xxMcuCfg_Init1'
      | sbobj.Groups(5).Signals.XData = [0 0.001 0.001 10]
      | sbobj.Groups(5).Signals.YData = [1 1 0 0]
      | sbobj.Groups(6).Name = 'Group 6'
      | sbobj.Groups(6).Signals.Name = 'call_GmT1xxMcuCfg_Init1'
      | sbobj.Groups(6).Signals.XData = [0 0.001 0.001 8]
      | sbobj.Groups(6).Signals.YData = [1 1 0 0]
      | sbobj.Groups(6).TimeRange = [0 8]
  call_GmT1xxMcuCfg_Init1 : Outport  Tag=STV Outport
  wires:
  FromWs/1 -> Demux/1
  Demux/1 -> call_GmT1xxMcuCfg_Init1/1

== system CM010A_GmT1xxMcuCfg/GmT1xxMcuCfg/CopyRight2 ==

== system CM010A_GmT1xxMcuCfg/GmT1xxMcuCfg/GmT1xxMcuCfgInit1 ==
  function : TriggerPort  TriggerType=function-call
  CopyRight2 : Subsystem  Description=|  mask(Copyright Information){none=on}
      | Copyright info block.                                               
      |                                                                     
      | Place copyright information at the top of every subsystem in design.
      mask prompts: none "No parameters"
      mask help: Place copyright information at the top of every subsystem in design.
      mask Display:
      | NxtrConf = 'Nexteer Confidential';
      | 
      | sys = bdroot; %handle for the current model ("system")
      | first = get_param(sys,'Created');
      | first = first(end-3:end);  %year is last four digits
      | 
      | last = get_param(sys,'LastModifiedDate');
      | if isempty(last)
      |     last = datestr(now,'yyyy');
      | else
      |     last = last(end-3:end);
      | end
      | 
      | if strcmp(first,last)
      |     fprintf('%s -- Copyright %s Nexteer',NxtrConf,first)
      | else
      |     fprintf('%s -- %s%s- %s Nexteer',NxtrConf,char(169),first,last)
      | end
  Register Initialization : Subsystem  Priority=10
      settings: AttributesFormatString=Priority: %<Priority>

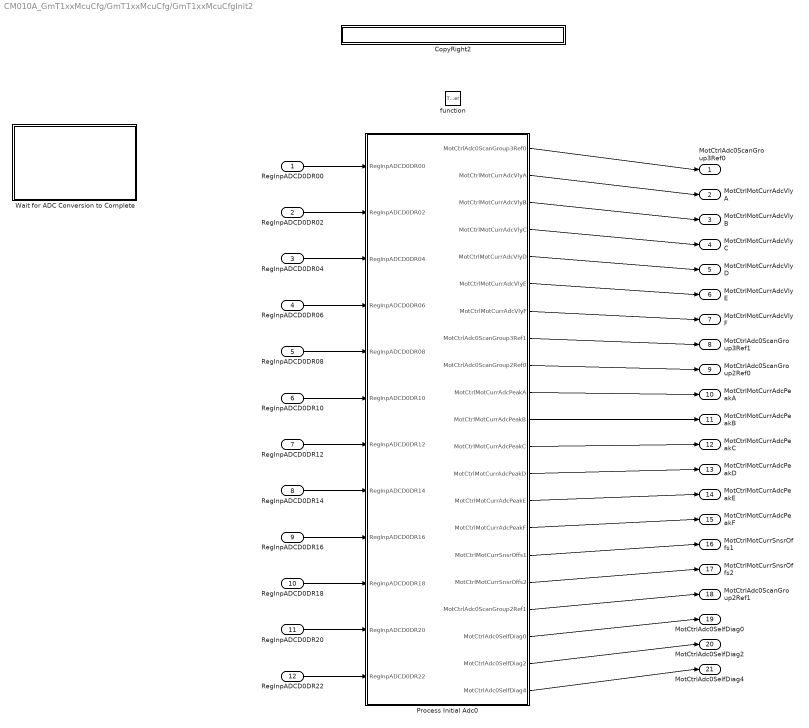
== system CM010A_GmT1xxMcuCfg/GmT1xxMcuCfg/GmT1xxMcuCfgInit2 ==
  RegInpADCD0DR00 : Inport  OutDataTypeStr=uint32
  RegInpADCD0DR02 : Inport  Port=2  OutDataTypeStr=uint32
  RegInpADCD0DR04 : Inport  Port=3  OutDataTypeStr=uint32
  RegInpADCD0DR06 : Inport  Port=4  OutDataTypeStr=uint32
  RegInpADCD0DR08 : Inport  Port=5  OutDataTypeStr=uint32
  RegInpADCD0DR10 : Inport  Port=6  OutDataTypeStr=uint32
  RegInpADCD0DR12 : Inport  Port=7  OutDataTypeStr=uint32
  RegInpADCD0DR14 : Inport  Port=8  OutDataTypeStr=uint32
  RegInpADCD0DR16 : Inport  Port=9  OutDataTypeStr=uint32
  RegInpADCD0DR18 : Inport  Port=10  OutDataTypeStr=uint32
  RegInpADCD0DR20 : Inport  Port=11  OutDataTypeStr=uint32
  RegInpADCD0DR22 : Inport  Port=12  OutDataTypeStr=uint32
  function : TriggerPort  TriggerType=function-call
  CopyRight2 : Subsystem  Description=|  mask(Copyright Information){none=on}
      | Copyright info block.                                               
      |                                                                     
      | Place copyright information at the top of every subsystem in design.
      mask prompts: none "No parameters"
      mask help: Place copyright information at the top of every subsystem in design.
      mask Display:
      | NxtrConf = 'Nexteer Confidential';
      | 
      | sys = bdroot; %handle for the current model ("system")
      | first = get_param(sys,'Created');
      | first = first(end-3:end);  %year is last four digits
      | 
      | last = get_param(sys,'LastModifiedDate');
      | if isempty(last)
      |     last = datestr(now,'yyyy');
      | else
      |     last = last(end-3:end);
      | end
      | 
      | if strcmp(first,last)
      |     fprintf('%s -- Copyright %s Nexteer',NxtrConf,first)
      | else
      |     fprintf('%s -- %s%s- %s Nexteer',NxtrConf,char(169),first,last)
      | end
  Process Initial Adc0 : Subsystem  RequirementInfo={'linktype_rmi_doors' '0000c472 (/ESG Group/FDD Module Requirements/EA4 Specific/CM300A_Adc0CfgAndUse)' '#CM300A_76' 'true' 'REQ: CM300A_76' '' ; 'linktype_rmi_doors' '0000c472 (/ESG Group/FDD Module Requirements/EA4 Specific/CM300A_Adc0CfgAndUse)' '#CM300A_81' 'true' 'REQ: CM300A_81' '' ; 'linktype_rmi_doors' '0000c472 (/ESG Group/FDD Module Requirements/EA4 Specific/CM300A_Adc0CfgAndUse)' '#CM300A_82' 'true' 'REQ: CM300A_82' '' } %GIDa_d862d82c_969a_40be_9cba_5dad28e4f649  Priority=20
      settings: AttributesFormatString=Priority: %<Priority>
  Wait for ADC Conversion to Complete : Subsystem  Priority=10
      settings: AttributesFormatString=Priority: %<Priority>
  MotCtrlAdc0ScanGroup3Ref0 : Outport
  MotCtrlMotCurrAdcVlyA : Outport  Port=2
  MotCtrlMotCurrAdcVlyB : Outport  Port=3
  MotCtrlMotCurrAdcVlyC : Outport  Port=4
  MotCtrlMotCurrAdcVlyD : Outport  Port=5
  MotCtrlMotCurrAdcVlyE : Outport  Port=6
  MotCtrlMotCurrAdcVlyF : Outport  Port=7
  MotCtrlAdc0ScanGroup3Ref1 : Outport  Port=8
  MotCtrlAdc0ScanGroup2Ref0 : Outport  Port=9
  MotCtrlMotCurrAdcPeakA : Outport  Port=10
  MotCtrlMotCurrAdcPeakB : Outport  Port=11
  MotCtrlMotCurrAdcPeakC : Outport  Port=12
  MotCtrlMotCurrAdcPeakD : Outport  Port=13
  MotCtrlMotCurrAdcPeakE : Outport  Port=14
  MotCtrlMotCurrAdcPeakF : Outport  Port=15
  MotCtrlMotCurrSnsrOffs1 : Outport  Port=16
  MotCtrlMotCurrSnsrOffs2 : Outport  Port=17
  MotCtrlAdc0ScanGroup2Ref1 : Outport  Port=18
  MotCtrlAdc0SelfDiag0 : Outport  Port=19
  MotCtrlAdc0SelfDiag2 : Outport  Port=20
  MotCtrlAdc0SelfDiag4 : Outport  Port=21
  wires:
  Process Initial Adc0/2(MotCtrlMotCurrAdcVlyA) -> MotCtrlMotCurrAdcVlyA/1
  Process Initial Adc0/3(MotCtrlMotCurrAdcVlyB) -> MotCtrlMotCurrAdcVlyB/1
  Process Initial Adc0/4(MotCtrlMotCurrAdcVlyC) -> MotCtrlMotCurrAdcVlyC/1
  Process Initial Adc0/5(MotCtrlMotCurrAdcVlyD) -> MotCtrlMotCurrAdcVlyD/1
  Process Initial Adc0/6(MotCtrlMotCurrAdcVlyE) -> MotCtrlMotCurrAdcVlyE/1
  Process Initial Adc0/7(MotCtrlMotCurrAdcVlyF) -> MotCtrlMotCurrAdcVlyF/1
  Process Initial Adc0/10(MotCtrlMotCurrAdcPeakA) -> MotCtrlMotCurrAdcPeakA/1
  Process Initial Adc0/11(MotCtrlMotCurrAdcPeakB) -> MotCtrlMotCurrAdcPeakB/1
  Process Initial Adc0/12(MotCtrlMotCurrAdcPeakC) -> MotCtrlMotCurrAdcPeakC/1
  Process Initial Adc0/13(MotCtrlMotCurrAdcPeakD) -> MotCtrlMotCurrAdcPeakD/1
  Process Initial Adc0/14(MotCtrlMotCurrAdcPeakE) -> MotCtrlMotCurrAdcPeakE/1
  Process Initial Adc0/15(MotCtrlMotCurrAdcPeakF) -> MotCtrlMotCurrAdcPeakF/1
  Process Initial Adc0/16(MotCtrlMotCurrSnsrOffs1) -> MotCtrlMotCurrSnsrOffs1/1
  Process Initial Adc0/17(MotCtrlMotCurrSnsrOffs2) -> MotCtrlMotCurrSnsrOffs2/1
  Process Initial Adc0/19(MotCtrlAdc0SelfDiag0) -> MotCtrlAdc0SelfDiag0/1
  Process Initial Adc0/20(MotCtrlAdc0SelfDiag2) -> MotCtrlAdc0SelfDiag2/1
  Process Initial Adc0/21(MotCtrlAdc0SelfDiag4) -> MotCtrlAdc0SelfDiag4/1
  RegInpADCD0DR00/1 -> Process Initial Adc0/1(RegInpADCD0DR00)
  RegInpADCD0DR02/1 -> Process Initial Adc0/2(RegInpADCD0DR02)
  RegInpADCD0DR04/1 -> Process Initial Adc0/3(RegInpADCD0DR04)
  RegInpADCD0DR06/1 -> Process Initial Adc0/4(RegInpADCD0DR06)
  RegInpADCD0DR08/1 -> Process Initial Adc0/5(RegInpADCD0DR08)
  RegInpADCD0DR10/1 -> Process Initial Adc0/6(RegInpADCD0DR10)
  RegInpADCD0DR12/1 -> Process Initial Adc0/7(RegInpADCD0DR12)
  RegInpADCD0DR14/1 -> Process Initial Adc0/8(RegInpADCD0DR14)
  RegInpADCD0DR16/1 -> Process Initial Adc0/9(RegInpADCD0DR16)
  RegInpADCD0DR18/1 -> Process Initial Adc0/10(RegInpADCD0DR18)
  RegInpADCD0DR20/1 -> Process Initial Adc0/11(RegInpADCD0DR20)
  RegInpADCD0DR22/1 -> Process Initial Adc0/12(RegInpADCD0DR22)
  Process Initial Adc0/8(MotCtrlAdc0ScanGroup3Ref1) -> MotCtrlAdc0ScanGroup3Ref1/1
  Process Initial Adc0/9(MotCtrlAdc0ScanGroup2Ref0) -> MotCtrlAdc0ScanGroup2Ref0/1
  Process Initial Adc0/1(MotCtrlAdc0ScanGroup3Ref0) -> MotCtrlAdc0ScanGroup3Ref0/1
  Process Initial Adc0/18(MotCtrlAdc0ScanGroup2Ref1) -> MotCtrlAdc0ScanGroup2Ref1/1

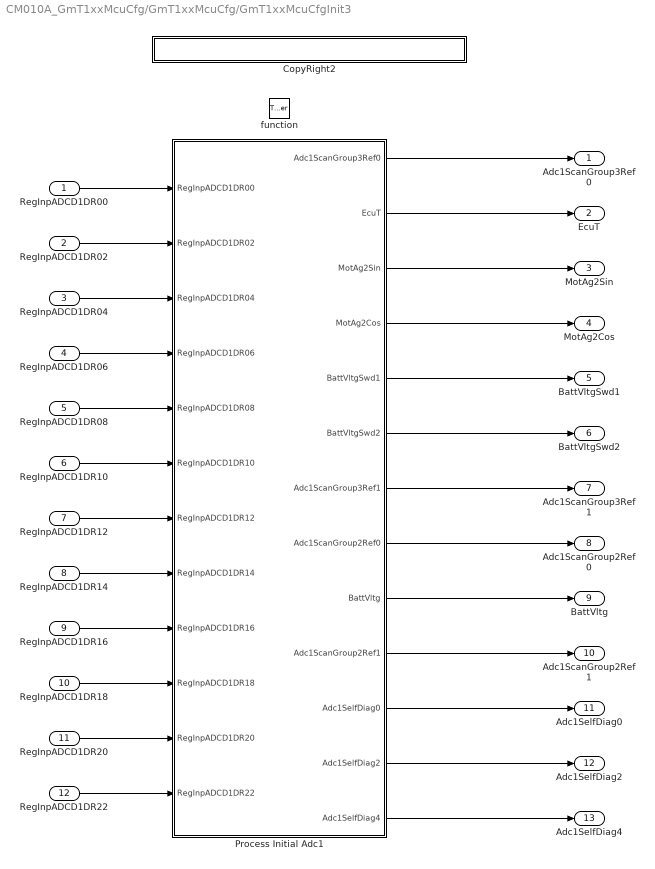
== system CM010A_GmT1xxMcuCfg/GmT1xxMcuCfg/GmT1xxMcuCfgInit3 ==
  RegInpADCD1DR00 : Inport  OutDataTypeStr=uint32
  RegInpADCD1DR02 : Inport  Port=2  OutDataTypeStr=uint32
  RegInpADCD1DR04 : Inport  Port=3  OutDataTypeStr=uint32
  RegInpADCD1DR06 : Inport  Port=4  OutDataTypeStr=uint32
  RegInpADCD1DR08 : Inport  Port=5  OutDataTypeStr=uint32
  RegInpADCD1DR10 : Inport  Port=6  OutDataTypeStr=uint32
  RegInpADCD1DR12 : Inport  Port=7  OutDataTypeStr=uint32
  RegInpADCD1DR14 : Inport  Port=8  OutDataTypeStr=uint32
  RegInpADCD1DR16 : Inport  Port=9  OutDataTypeStr=uint32
  RegInpADCD1DR18 : Inport  Port=10  OutDataTypeStr=uint32
  RegInpADCD1DR20 : Inport  Port=11  OutDataTypeStr=uint32
  RegInpADCD1DR22 : Inport  Port=12  OutDataTypeStr=uint32
  function : TriggerPort  TriggerType=function-call
  CopyRight2 : Subsystem  Description=|  mask(Copyright Information){none=on}
      | Copyright info block.                                               
      |                                                                     
      | Place copyright information at the top of every subsystem in design.
      mask prompts: none "No parameters"
      mask help: Place copyright information at the top of every subsystem in design.
      mask Display:
      | NxtrConf = 'Nexteer Confidential';
      | 
      | sys = bdroot; %handle for the current model ("system")
      | first = get_param(sys,'Created');
      | first = first(end-3:end);  %year is last four digits
      | 
      | last = get_param(sys,'LastModifiedDate');
      | if isempty(last)
      |     last = datestr(now,'yyyy');
      | else
      |     last = last(end-3:end);
      | end
      | 
      | if strcmp(first,last)
      |     fprintf('%s -- Copyright %s Nexteer',NxtrConf,first)
      | else
      |     fprintf('%s -- %s%s- %s Nexteer',NxtrConf,char(169),first,last)
      | end
  Process Initial Adc1 : Subsystem  RequirementInfo={'linktype_rmi_doors' '0000c472 (/ESG Group/FDD Module Requirements/EA4 Specific/CM300A_Adc0CfgAndUse)' '#CM300A_76' 'true' 'REQ: CM300A_76' '' ; 'linktype_rmi_doors' '0000c472 (/ESG Group/FDD Module Requirements/EA4 Specific/CM300A_Adc0CfgAndUse)' '#CM300A_81' 'true' 'REQ: CM300A_81' '' ; 'linktype_rmi_doors' '0000c472 (/ESG Group/FDD Module Requirements/EA4 Specific/CM300A_Adc0CfgAndUse)' '#CM300A_82' 'true' 'REQ: CM300A_82' '' } %GIDa_376048c3_94d2_40f9_9974_227dea3c5b4f  Priority=40
      settings: AttributesFormatString=Priority: %<Priority>
  Adc1ScanGroup3Ref0 : Outport
  EcuT : Outport  Port=2
  MotAg2Sin : Outport  Port=3
  MotAg2Cos : Outport  Port=4
  BattVltgSwd1 : Outport  Port=5
  BattVltgSwd2 : Outport  Port=6
  Adc1ScanGroup3Ref1 : Outport  Port=7
  Adc1ScanGroup2Ref0 : Outport  Port=8
  BattVltg : Outport  Port=9
  Adc1ScanGroup2Ref1 : Outport  Port=10
  Adc1SelfDiag0 : Outport  Port=11
  Adc1SelfDiag2 : Outport  Port=12
  Adc1SelfDiag4 : Outport  Port=13
  wires:
  Process Initial Adc1/2(EcuT) -> EcuT/1
  Process Initial Adc1/3(MotAg2Sin) -> MotAg2Sin/1
  Process Initial Adc1/4(MotAg2Cos) -> MotAg2Cos/1
  Process Initial Adc1/5(BattVltgSwd1) -> BattVltgSwd1/1
  Process Initial Adc1/6(BattVltgSwd2) -> BattVltgSwd2/1
  Process Initial Adc1/9(BattVltg) -> BattVltg/1
  Process Initial Adc1/11(Adc1SelfDiag0) -> Adc1SelfDiag0/1
  Process Initial Adc1/12(Adc1SelfDiag2) -> Adc1SelfDiag2/1
  Process Initial Adc1/13(Adc1SelfDiag4) -> Adc1SelfDiag4/1
  RegInpADCD1DR00/1 -> Process Initial Adc1/1(RegInpADCD1DR00)
  RegInpADCD1DR02/1 -> Process Initial Adc1/2(RegInpADCD1DR02)
  RegInpADCD1DR04/1 -> Process Initial Adc1/3(RegInpADCD1DR04)
  RegInpADCD1DR06/1 -> Process Initial Adc1/4(RegInpADCD1DR06)
  RegInpADCD1DR08/1 -> Process Initial Adc1/5(RegInpADCD1DR08)
  RegInpADCD1DR10/1 -> Process Initial Adc1/6(RegInpADCD1DR10)
  RegInpADCD1DR12/1 -> Process Initial Adc1/7(RegInpADCD1DR12)
  RegInpADCD1DR14/1 -> Process Initial Adc1/8(RegInpADCD1DR14)
  RegInpADCD1DR16/1 -> Process Initial Adc1/9(RegInpADCD1DR16)
  RegInpADCD1DR18/1 -> Process Initial Adc1/10(RegInpADCD1DR18)
  RegInpADCD1DR20/1 -> Process Initial Adc1/11(RegInpADCD1DR20)
  RegInpADCD1DR22/1 -> Process Initial Adc1/12(RegInpADCD1DR22)
  Process Initial Adc1/1(Adc1ScanGroup3Ref0) -> Adc1ScanGroup3Ref0/1
  Process Initial Adc1/7(Adc1ScanGroup3Ref1) -> Adc1ScanGroup3Ref1/1
  Process Initial Adc1/8(Adc1ScanGroup2Ref0) -> Adc1ScanGroup2Ref0/1
  Process Initial Adc1/10(Adc1ScanGroup2Ref1) -> Adc1ScanGroup2Ref1/1
